simulink model "DTU_Topology_Rural"  (R2023b)
settings: Solver=ode4  StartTime=0.0  StopTime=stoptime  FixedStep=Ts  RelTol=1e-3
PreLoadFcn:
  | Ts=1e-4;load('RuralCase_11052022_12052022_Data_with_ParThreads_Final.mat');run('line_parameters.m');run('Grid_Parameters_3ph.m');
PostLoadFcn:
  | Ts=1e-4;load('RuralCase_11052022_12052022_Data_with_ParThreads_Final.mat');run('line_parameters.m');run('Grid_Parameters_3ph.m');
InitFcn:
  | Ts=1e-4;load('RuralCase_11052022_12052022_Data_with_ParThreads_Final.mat');run('line_parameters.m');run('Grid_Parameters_3ph.m');
StartFcn:
  | Ts=1e-4;load('RuralCase_11052022_12052022_Data_with_ParThreads_Final.mat');run('line_parameters.m');run('Grid_Parameters_3ph.m');
values from neighbouring files (symbols this model uses):
  datastart = 1    [Grid_Parameters_3ph.m]
  datastop = 21556    [Grid_Parameters_3ph.m]
  DTUsignconv = -1000    [Grid_Parameters_3ph.m]
  fnom = 50    [Grid_Parameters_3ph.m]    (also in line_parameters.m)
  line_param = struct()    [line_parameters.m]
  Time = cumsum([0;ones(stoptime,1)])    [Grid_Parameters_3ph.m]
  timestep_meas_data = 1    [Grid_Parameters_3ph.m]
  Vnom = 400    [Grid_Parameters_3ph.m]
undefined symbols (not defined in the file or in its folder): another_event_name, data, j, my_event_name, Newton, Raphson, t_factor
libraries: spsSeriesRLCBranchLib x126, spsGroundLib x71, spsThreePhaseSineGeneratorLib x42, spsControlledCurrentSourceLib x39, spsThreePhaseVIMeasurementLib x26, spsMeanLib x24, spsPowerLib x14, spsMutualInductanceLib x7, rtlab x3, powerlib_meascontrol x3, spsControlledVoltageSourceLib x3, spsThreePhaseSourceLib x1
(part 1 of 5)
Description:
  | Model of a simple control system for use iin training.
settings Model: VariantFading=off  Creator=Alex  LastModifiedBy=obus
settings SolverCC: AlgebraicLoopSolver=TrustRegion  AutoInsertRateTranBlk=on
settings DataIOCC: LimitDataPoints=on  SaveFormat=Array  SignalLoggingSaveFormat=ModelDataLogs  SaveOutput=off  SaveTime=off  ReturnWorkspaceOutputs=off  SignalLoggingName=sigsOut
settings OptimizationCC: BlockReduction=off  BooleanDataType=off  OptimizeBlockIOStorage=off  BufferReuse=off  GlobalBufferReuse=off  ExpressionFolding=off  LocalBlockOutputs=off  InitFltsAndDblsToZero=on  LifeSpan=inf  OptimizeDataStoreBuffers=off  BusAssignmentInplaceUpdate=off
settings DebuggingCC: SaveWithParameterizedLinksMsg=none  UnderspecifiedInitializationDetection=Classic  MergeDetectMultiDrivingBlocksExec=none  SignalResolutionControl=TryResolveAllWithWarning  MultiTaskDSMMsg=warning  MultiTaskCondExecSysMsg=none  FcnCallInpInsideContextMsg=warning  UnconnectedInputMsg=warning  UnconnectedOutputMsg=warning  UnconnectedLineMsg=warning  SFUnexpectedBacktrackingDiag=warning  SFNoUnconditionalDefaultTransitionDiag=warning  SFExecutionAtInitializationDiag=none  ArithmeticOperatorsInVariantConditions=warning
settings HardwareCC: ProdBitPerPointer=32  ProdBitPerSizeT=32  ProdBitPerPtrDiffT=32  ProdLargestAtomicFloat=None  ProdIntDivRoundTo=Undefined  ProdEndianess=Unspecified  ProdWordSize=32  ProdHWDeviceType=32-bit Generic  TargetUnknown=on
settings ModelReferenceCC: EnableRefExpFcnMdlSchedulingChecks=on  PropagateSignalLabelsOutOfModel=off
settings SFSimCC: SimUseLocalCustomCode=off  CustomCodeUndefinedFunction=UseInterfaceOnly
settings RTWCC: RTWUseLocalCustomCode=off  DLArmComputeVersion=19.05
settings CodeAppCC: StateflowObjectComments=on
settings GRTTargetCC: TargetFcnLib=ansi_tfl_tmw.mat  TargetLangStandard=C89/C90 (ANSI)  CombineOutputUpdateFcns=off  GRTInterface=on
settings ConfigComp: CovMetricSettings=dw  CovSaveCumulativeToWorkspaceVar=on  CovSaveSingleToWorkspaceVar=on  CovExternalEMLEnable=off

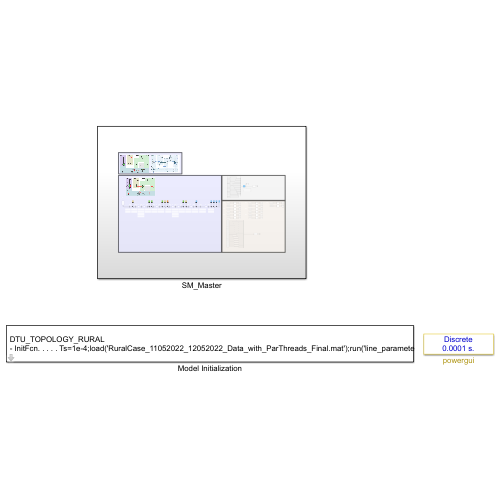
[thumbnail: Simulink's stored preview of the top-level diagram]
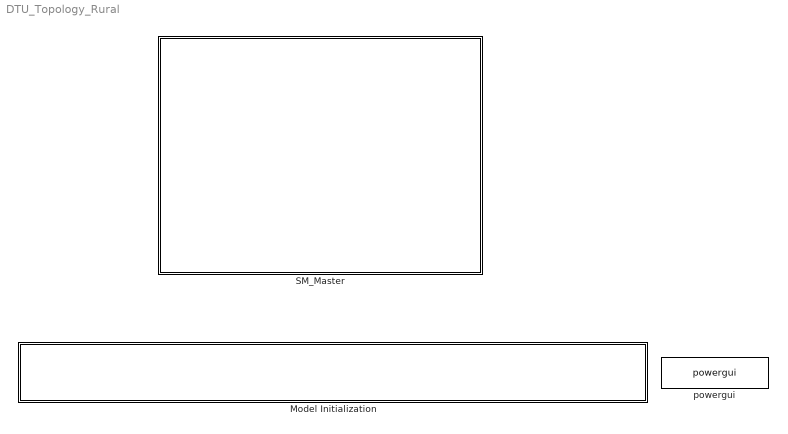
== system DTU_Topology_Rural ==
  Model Initialization : Subsystem  mask(Model Functions){InitFcnX=Ts=1e-4;load('RuralCase_11052022_12052022_Data_with_ParThreads_Final.mat');run('line_parameters.m');run('Grid_Parameters_3ph.m');, prel=on, posl=on, inif=on, strf=on}
      mask prompts: InitFcnX "Initialisation"; prel "Preload Function"; posl "PostLoad Function"; inif "InitFcn"; strf "StartFcn"
      mask init:
      | currentBlock = gcb;
      | root = bdroot(currentBlock);
      | 
      | if ~strcmp(get_param(root,'BlockDiagramType'),'library')
      |     if prel==1
      |         set_param(root, 'PreLoadFcn', InitFcnX);
      |     else
      |         set_param(root, 'PreLoadFcn', '');
      |     end
      |     if inif==1
      |         set_param(root, 'InitFcn', InitFcnX);
      |     else
      |         set_param(root, 'InitFcn', '');
      |     end
      |     if strf==1
      |         set_param(root, 'StartFcn', InitFcnX);
      |     else
      |         set_param(root, 'StartFcn', '');
      |     end
      |     if posl==1
      |         set_param(root, 'PostLoadFcn', InitFcnX);
      |     else
      |         set_param(root, 'PostLoadFcn', '');
      |     end
      | end
      | 
      | pos = get_param(currentBlock, 'Position');
      | width = pos(3) - pos(1); height = pos(4) - pos(2);
      | txt = [ upper(root) '\n' '- InitFcn. . . . . '  get_param(root, 'InitFcn') ];
      settings: CopyFcn=set_param(gcb,'LinkStatus','none')
      mask Display: text(5, height*0.5, txt, 'horizontalAlignment', 'left', 'verticalAlignment', 'middle') ;
  SM_Master : Subsystem
  powergui : sps_lib/powergui  Priority=2  SimulationMode=Discrete  SampleTime=Ts  frequency=60  Iterations=50  frequencyindice=50  Pbase=100e6  ErrMax=1e-4  UnitsV=V  UnitsW=kW  buscounter=0  FunctionMessages=off  echomessages=off  EnableUseOfTLC=off  CurrentSourceSwitches=off  DisableSnubberDevices=off  DisableRonSwitches=off  DisableVfSwitches=off  DisplayEquations=off  AutomaticDiscreteSolvers=off  SolverType=Tustin  Interpol=off  ExternalGateDelay=off  methode=off  Ts=0  x0status=steady  SPID=off  SwTol=0  HookPort=off  NonlinearTolerance=0  nMaxIteration=15  ContinueOnMaxIteration=off  RestoreLinks=warning  ResistiveCurrentMeasurement=off  Frange=logspace(0,3,50)  Ylog=off  Xlog=off  ShowGrid=off  save=off  variable=ZData  structure=0  ZoomFFT=on  StartTime=0.0  cycles=1  DisplayStyle=1  fundamental=60  FreqAxis=off  MaxFrequency=1000  frequencyindicesteady=1  RmsSteady=2  display=off

== system DTU_Topology_Rural/Model Initialization ==

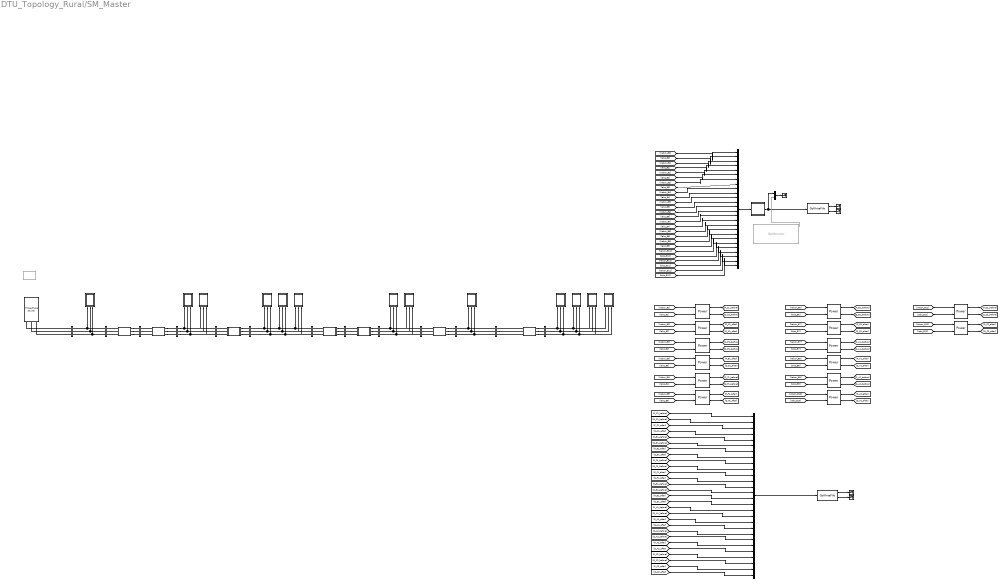
== system DTU_Topology_Rural/SM_Master ==
  note: 700m
  note: DTU SYSLAB Rural Topology
  note: Topology
  note: delta C1
  note: RT-Signals
  note: delta F1
  note: ΔP & ΔQ calculations
  note: delta E1
  note: Iabc_B0
  note: Vabcn_B0
  note: Vabcn_B1
  note: Iabc_B1
  note: Vabcn_B2
  note: Iabc_B2
  note: Vabcn_B3
  note: Iabc_B3
  note: Iabc_B4
  note: Vabcn_B4
  note: Iabc_B5
  note: Vabcn_B5
  note: Vabcn_B6
  note: Iabc_B6
  note: Iabc_B7
  note: Vabcn_B7
  note: Iabc_B8
  note: Vabcn_B8
  note: Vabcn_B9
  note: Iabc_B9
  note: Iabc_B10
  note: Vabcn_B10
  note: Vabcn_B12
  note: Iabc_B12
  note: delta A1
  note: delta A2
  note: delta B1
  note: delta C2
  note: 2:4
      | '117-2_Grid_phaseA_Voltage',
      | '117-2_Grid_phaseB_Voltage',
      | '117-2_Grid_phaseC_Voltage'
  note: 5:7
      | '117-2_Grid_phaseA_Current',
      | '117-2_Grid_phaseB_Current',
      | '117-2_Grid_phaseC_Current'
  note: 8:10
      | '117-2_Cable1_phaseA_Voltage',
      | '117-2_Cable1_phaseB_Voltage',
      | '117-2_Cable1_phaseC_Voltage'
  note: 11:13
      | '117-2_Cable1_phaseA_Current',
      | '117-2_Cable1_phaseB_Current',
      | '117-2_Cable1_phaseC_Current'
  note: 17:19
      | '319-3_C1 to 117-2_phaseA_Current',
      | '319-3_C1 to 117-2_phaseB_Current',
      | '319-3_C1 to 117-2_phaseC_Current'
  note: 14:16
      | '319-3_C1 to 117-2_phaseA_Voltage',
      | '319-3_C1 to 117-2_phaseB_Voltage',
      | '319-3_C1 to 117-2_phaseC_Voltage'
  note: same as 17:19
      | '319-3_E1 to 716-2_phaseA_Current',
      | '319-3_E1 to 716-2_phaseB_Current',
      | '319-3_E1 to 716-2_phaseC_Current'
  note: same as 14:16
      | '319-3_E1 to 716-2_phaseA_Voltage',
      | '319-3_E1 to 716-2_phaseB_Voltage',
      | '319-3_E1 to 716-2_phaseC_Voltage'
  note: 23:25
      | '716-2_CableE1_phaseA_Current',
      | '716-2_CableE1_phaseB_Current',
      | '716-2_CableE1_phaseC_Current'
  note: 20:22
      | '716-2_CableE1_phaseA_Voltage',
      | '716-2_CableE1_phaseB_Voltage',
      | '716-2_CableE1_phaseC_Voltage'
  note: 26:28
      | '716-2_Cable F1_phaseA_Voltage',
      | '716-2_Cable F1_phaseB_Voltage',
      | '716-2_Cable F1_phaseC_Voltage'
  note: 29:31
      | '716-2_Cable F1_phaseA_Current',
      | '716-2_Cable F1_phaseB_Current',
      | '716-2_Cable F1_phaseC_Current'
  note: 35:37
      | '715-2_CableF1_phaseA_Current',
      | '715-2_CableF1_phaseB_Current',
      | '715-2_CableF1_phaseC_Current'
  note: 32:34
      | '715-2_CableF1_phaseA_Voltage',
      | '715-2_CableF1_phaseB_Voltage',
      | '715-2_CableF1_phaseC_Voltage'
  note: 38:40
      | '715-2_CableB1_phaseA_Voltage',
      | '715-2_CableB1_phaseB_Voltage',
      | '715-2_CableB1_phaseC_Voltage'
  note: 41:43
      | '715-2_CableB1_phaseA_Current',
      | '715-2_CableB1_phaseB_Current',
      | '715-2_CableB1_phaseC_Current'
  note: 47:49
      | '319-3_B1 to 715-2_phaseA_Current',
      | '319-3_B1 to 715-2_phaseB_Current',
      | '319-3_B1 to 715-2_phaseC_Current'
  note: 44:46
      | '319-3_B1 to 715-2_phaseA_Voltage',
      | '319-3_B1 to 715-2_phaseB_Voltage',
      | '319-3_B1 to 715-2_phaseC_Voltage'
  note: same as 47:49
      | '319-3_A1 to 319-2_phaseA_Current',
      | '319-3_A1 to 319-2_phaseB_Current',
      | '319-3_A1 to 319-2_phaseC_Current'
  note: same as 44:46
      | '319-3_A1 to 319-2_phaseA_Voltage',
      | '319-3_A1 to 319-2_phaseB_Voltage',
      | '319-3_A1 to 319-2_phaseC_Voltage'
  note: 53:55
      | '319-2_Cable1_phaseA_Current',
      | '319-2_Cable1_phaseB_Current',
      | '319-2_Cable1_phaseC_Current'
  note: 50:52
      | '319-2_Cable1_phaseA_Voltage',
      | '319-2_Cable1_phaseB_Voltage',
      | '319-2_Cable1_phaseC_Voltage'
  note: 59:61
      | '319-2_Cable2_phaseA_Current',
      | '319-2_Cable2_phaseB_Current',
      | '319-2_Cable2_phaseC_Current'
  note: 56:58
      | '319-2_Cable2_phaseA_Voltage',
      | '319-2_Cable2_phaseB_Voltage',
      | '319-2_Cable2_phaseC_Voltage'
  note: 68:70
      | '319-3_C2 to 117-2_phaseA_Voltage',
      | '319-3_C2 to 117-2_phaseB_Voltage',
      | '319-3_C2 to 117-2_phaseC_Voltage'
  note: 71:73
      | '319-3_C2 to 117-2_phaseA_Current',
      | '319-3_C2 to 117-2_phaseB_Current',
      | '319-3_C2 to 117-2_phaseC_Current'
  note: 62:64
      | '319-3_A2 to 319-2_phaseA_Voltage',
      | '319-3_A2 to 319-2_phaseB_Voltage',
      | '319-3_A2 to 319-2_phaseC_Voltage'
  note: 65:67
      | '319-3_A2 to 319-2_phaseA_Current',
      | '319-3_A2 to 319-2_phaseB_Current',
      | '319-3_A2 to 319-2_phaseC_Current'
  note: 77:79
      | '117-2_Cable2_phaseA_Current',
      | '117-2_Cable2_phaseB_Current',
      | '117-2_Cable2_phaseC_Current'
  note: 74:76
      | '117-2_Cable2_phaseA_Voltage',
      | '117-2_Cable2_phaseB_Voltage',
      | '117-2_Cable2_phaseC_Voltage'
  note: 450m
  note: 330m
  note: 350m
  note: 25m
  note: 25m
  note: 700m
  note: Iabc_B11
  note: Vabcn_B11
  B0_n : spsThreePhaseVIMeasurementLib/Three-Phase V-I Measurement  VoltageMeasurement=phase-to-ground  SetLabelV=on  LabelV=Vabcn_B0  Vpu=off  VpuLL=off  CurrentMeasurement=yes  SetLabelI=on  LabelI=Iabc_B0  Ipu=off  Pbase=900e6  Vbase=400  OutputType=Complex  PhasorSimulation=off  PSBequivalent=0
  B10_n : spsThreePhaseVIMeasurementLib/Three-Phase V-I Measurement  VoltageMeasurement=phase-to-ground  SetLabelV=on  LabelV=Vabcn_B10  Vpu=off  VpuLL=off  CurrentMeasurement=yes  SetLabelI=on  LabelI=Iabc_B10  Ipu=off  Pbase=900e6  Vbase=400  OutputType=Complex  PhasorSimulation=off  PSBequivalent=0
  B11_n : spsThreePhaseVIMeasurementLib/Three-Phase V-I Measurement  VoltageMeasurement=phase-to-ground  SetLabelV=on  LabelV=Vabcn_B11  Vpu=off  VpuLL=off  CurrentMeasurement=yes  SetLabelI=on  LabelI=Iabc_B11  Ipu=off  Pbase=900e6  Vbase=400  OutputType=Complex  PhasorSimulation=off  PSBequivalent=0
  B12_n : spsThreePhaseVIMeasurementLib/Three-Phase V-I Measurement  VoltageMeasurement=phase-to-ground  SetLabelV=on  LabelV=Vabcn_B12  Vpu=off  VpuLL=off  CurrentMeasurement=yes  SetLabelI=on  LabelI=Iabc_B12  Ipu=off  Pbase=900e6  Vbase=400  OutputType=Complex  PhasorSimulation=off  PSBequivalent=0
  B1_n : spsThreePhaseVIMeasurementLib/Three-Phase V-I Measurement  VoltageMeasurement=phase-to-ground  SetLabelV=on  LabelV=Vabcn_B1  Vpu=off  VpuLL=off  CurrentMeasurement=yes  SetLabelI=on  LabelI=Iabc_B1  Ipu=off  Pbase=900e6  Vbase=400  OutputType=Complex  PhasorSimulation=off  PSBequivalent=0
  B2_n : spsThreePhaseVIMeasurementLib/Three-Phase V-I Measurement  VoltageMeasurement=phase-to-ground  SetLabelV=on  LabelV=Vabcn_B2  Vpu=off  VpuLL=off  CurrentMeasurement=yes  SetLabelI=on  LabelI=Iabc_B2  Ipu=off  Pbase=900e6  Vbase=400  OutputType=Complex  PhasorSimulation=off  PSBequivalent=0
  B3_n : spsThreePhaseVIMeasurementLib/Three-Phase V-I Measurement  VoltageMeasurement=phase-to-ground  SetLabelV=on  LabelV=Vabcn_B3  Vpu=off  VpuLL=off  CurrentMeasurement=yes  SetLabelI=on  LabelI=Iabc_B3  Ipu=off  Pbase=900e6  Vbase=400  OutputType=Complex  PhasorSimulation=off  PSBequivalent=0
  B4_n : spsThreePhaseVIMeasurementLib/Three-Phase V-I Measurement  VoltageMeasurement=phase-to-ground  SetLabelV=on  LabelV=Vabcn_B4  Vpu=off  VpuLL=off  CurrentMeasurement=yes  SetLabelI=on  LabelI=Iabc_B4  Ipu=off  Pbase=900e6  Vbase=400  OutputType=Complex  PhasorSimulation=off  PSBequivalent=0
  B5_n : spsThreePhaseVIMeasurementLib/Three-Phase V-I Measurement  VoltageMeasurement=phase-to-ground  SetLabelV=on  LabelV=Vabcn_B5  Vpu=off  VpuLL=off  CurrentMeasurement=yes  SetLabelI=on  LabelI=Iabc_B5  Ipu=off  Pbase=900e6  Vbase=400  OutputType=Complex  PhasorSimulation=off  PSBequivalent=0
  B6_n : spsThreePhaseVIMeasurementLib/Three-Phase V-I Measurement  VoltageMeasurement=phase-to-ground  SetLabelV=on  LabelV=Vabcn_B6  Vpu=off  VpuLL=off  CurrentMeasurement=yes  SetLabelI=on  LabelI=Iabc_B6  Ipu=off  Pbase=900e6  Vbase=400  OutputType=Complex  PhasorSimulation=off  PSBequivalent=0
  B7_n : spsThreePhaseVIMeasurementLib/Three-Phase V-I Measurement  VoltageMeasurement=phase-to-ground  SetLabelV=on  LabelV=Vabcn_B7  Vpu=off  VpuLL=off  CurrentMeasurement=yes  SetLabelI=on  LabelI=Iabc_B7  Ipu=off  Pbase=900e6  Vbase=400  OutputType=Complex  PhasorSimulation=off  PSBequivalent=0
  B8_n : spsThreePhaseVIMeasurementLib/Three-Phase V-I Measurement  VoltageMeasurement=phase-to-ground  SetLabelV=on  LabelV=Vabcn_B8  Vpu=off  VpuLL=off  CurrentMeasurement=yes  SetLabelI=on  LabelI=Iabc_B8  Ipu=off  Pbase=900e6  Vbase=400  OutputType=Complex  PhasorSimulation=off  PSBequivalent=0
  B9_n : spsThreePhaseVIMeasurementLib/Three-Phase V-I Measurement  VoltageMeasurement=phase-to-ground  SetLabelV=on  LabelV=Vabcn_B9  Vpu=off  VpuLL=off  CurrentMeasurement=yes  SetLabelI=on  LabelI=Iabc_B9  Ipu=off  Pbase=900e6  Vbase=400  OutputType=Complex  PhasorSimulation=off  PSBequivalent=0
  Cable A1 No parallel cap : Subsystem  mask(ZHAW_Config){fNom=fnom, length=line_param.A1.length}
      mask prompts: fNom "Nominal frequency (Hz)"; length "Length (km)"
      mask Display:
      | patch([20 20 80 80], [0 20 20 0])
      | patch([0 0 20 20], [7 13 13 7])
      | patch([80 80 100 100], [7 13 13 7])
      | 
      | patch([20 20 80 80], [40 60 60 40])
      | patch([0 0 20 20], [47 53 53 47])
      | patch([80 80 100 100], [47 53 53 47])
      | 
      | patch([20 20 80 80], [80 100 100 80])
      | patch([0 0 20 20], [87 93 93 87])
      | patch([80 80 100 100], [87 93 93 87])
  Cable A2 No parallel cap : Subsystem  mask(ZHAW_Config){fNom=fnom, length=line_param.A2.length}
      mask prompts: fNom "Nominal frequency (Hz)"; length "Length (km)"
      mask Display:
      | patch([20 20 80 80], [0 20 20 0])
      | patch([0 0 20 20], [7 13 13 7])
      | patch([80 80 100 100], [7 13 13 7])
      | 
      | patch([20 20 80 80], [40 60 60 40])
      | patch([0 0 20 20], [47 53 53 47])
      | patch([80 80 100 100], [47 53 53 47])
      | 
      | patch([20 20 80 80], [80 100 100 80])
      | patch([0 0 20 20], [87 93 93 87])
      | patch([80 80 100 100], [87 93 93 87])
  Cable B1 No parallel cap : Subsystem  mask(ZHAW_Config){fNom=fnom, length=line_param.B1.length}
      mask prompts: fNom "Nominal frequency (Hz)"; length "Length (km)"
      mask Display:
      | patch([20 20 80 80], [0 20 20 0])
      | patch([0 0 20 20], [7 13 13 7])
      | patch([80 80 100 100], [7 13 13 7])
      | 
      | patch([20 20 80 80], [40 60 60 40])
      | patch([0 0 20 20], [47 53 53 47])
      | patch([80 80 100 100], [47 53 53 47])
      | 
      | patch([20 20 80 80], [80 100 100 80])
      | patch([0 0 20 20], [87 93 93 87])
      | patch([80 80 100 100], [87 93 93 87])
  Cable C1 No parallel cap : Subsystem  mask(ZHAW_Config){fNom=fnom, length=line_param.C1.length}
      mask prompts: fNom "Nominal frequency (Hz)"; length "Length (km)"
      mask Display:
      | patch([20 20 80 80], [0 20 20 0])
      | patch([0 0 20 20], [7 13 13 7])
      | patch([80 80 100 100], [7 13 13 7])
      | 
      | patch([20 20 80 80], [40 60 60 40])
      | patch([0 0 20 20], [47 53 53 47])
      | patch([80 80 100 100], [47 53 53 47])
      | 
      | patch([20 20 80 80], [80 100 100 80])
      | patch([0 0 20 20], [87 93 93 87])
      | patch([80 80 100 100], [87 93 93 87])
  Cable C2 No parallel cap : Subsystem  mask(ZHAW_Config){fNom=fnom, length=line_param.C2.length}
      mask prompts: fNom "Nominal frequency (Hz)"; length "Length (km)"
      mask Display:
      | patch([20 20 80 80], [0 20 20 0])
      | patch([0 0 20 20], [7 13 13 7])
      | patch([80 80 100 100], [7 13 13 7])
      | 
      | patch([20 20 80 80], [40 60 60 40])
      | patch([0 0 20 20], [47 53 53 47])
      | patch([80 80 100 100], [47 53 53 47])
      | 
      | patch([20 20 80 80], [80 100 100 80])
      | patch([0 0 20 20], [87 93 93 87])
      | patch([80 80 100 100], [87 93 93 87])
  Cable E1 No parallel cap : Subsystem  mask(ZHAW_Config){fNom=fnom, length=line_param.E1.length}
      mask prompts: fNom "Nominal frequency (Hz)"; length "Length (km)"
      mask Display:
      | patch([20 20 80 80], [0 20 20 0])
      | patch([0 0 20 20], [7 13 13 7])
      | patch([80 80 100 100], [7 13 13 7])
      | 
      | patch([20 20 80 80], [40 60 60 40])
      | patch([0 0 20 20], [47 53 53 47])
      | patch([80 80 100 100], [47 53 53 47])
      | 
      | patch([20 20 80 80], [80 100 100 80])
      | patch([0 0 20 20], [87 93 93 87])
      | patch([80 80 100 100], [87 93 93 87])
  Cable F1 No parallel cap : Subsystem  mask(ZHAW_Config){fNom=fnom, length=line_param.F1.length}
      mask prompts: fNom "Nominal frequency (Hz)"; length "Length (km)"
      mask Display:
      | patch([20 20 80 80], [0 20 20 0])
      | patch([0 0 20 20], [7 13 13 7])
      | patch([80 80 100 100], [7 13 13 7])
      | 
      | patch([20 20 80 80], [40 60 60 40])
      | patch([0 0 20 20], [47 53 53 47])
      | patch([80 80 100 100], [47 53 53 47])
      | 
      | patch([20 20 80 80], [80 100 100 80])
      | patch([0 0 20 20], [87 93 93 87])
      | patch([80 80 100 100], [87 93 93 87])
  External Grid 400V : spsThreePhaseSourceLib/Three-Phase Source  InternalConnection=Yg  VoltagePhases=off  Voltage=400  PhaseAngle=0  Voltage_phases=[400 400 400]/sqrt(3)*1.00006  PhaseAngles_phases=[0 -120 +120]  Frequency=50  NonIdealSource=on  SpecifyImpedance=on  Resistance=400^2/10e6/10  Inductance=400^2/10e6/(2*pi*50)  ShortCircuitLevel=60e6  BaseVoltage=400  XRratio=1/0.1  BusType=swing  Pref=0  Qref=0  Prefabc=[10e3, 10e3, 10e3]  Qrefabc=[0, 0, 0]  Qmin=-Inf  Qmax=Inf
  Mux2 : Mux  Inputs=2
  Mux3 : Mux  Inputs=3*ones(1,26)
  Mux5 : Mux  Inputs=3 * ones(1,28)
  OpMonitor : rtlab/Monitoring/OpMonitor  Commented=on  compute_time=on  real_step=on  idle_time=on  nb_overruns=on  user_time=off  user_name=my_event_name,another_event_name
      settings: SourceProductName=RT-LAB
  OpWriteFile : rtlab/DataLogging/OpWriteFile  Static_File=on  varname=DTU_Rural_Case_x_UI  Filename=DTU_Rural_Case_x_UI.mat  rtpath='./'  nrtpath='.\'  Acq_Group=26  file_size=[500e6]  write_offline=on  Sim_Mode=off  Nb_Samples=stoptime  Buffer_size=1000000
      settings: SourceProductName=RT-LAB  Decimation=10000
  OpWriteFile1 : rtlab/DataLogging/OpWriteFile  Static_File=on  varname=DTU_Rural_Case_x_PQ  Filename=DTU_Rural_Case_x_PQ.mat  rtpath='./'  nrtpath='.\'  Acq_Group=27  file_size=[500e6]  write_offline=on  Sim_Mode=off  Nb_Samples=stoptime  Buffer_size=1000000
      settings: SourceProductName=RT-LAB  Decimation=10000
  Power{,1..13} (14 alike) : spsPowerLib/Power  Freq=50  Vinit=[1, 0]  Iinit=[1, 0]  Ts=0
  Terminator{,1..4} (5 alike) : Terminator
  TrueRMS 1 : Subsystem  AncestorBlock=powerlib_meascontrol/Measurements/RMS/TrueRMS
  Uncontrollable EVSE 4 : Subsystem
  Uncontrollable EVSE 5 : Subsystem
  Uncontrollable EVSE 6 : Subsystem
  Uncontrollable EVSE 7 : Subsystem
  Uncontrollable EVSE V2G & EVSE SYSLAB : Subsystem
  Uncontrollable PV 117 : Subsystem
  Uncontrollable PV 319 : Subsystem
  Uncontrollable PV 715 : Subsystem
  Uncontrollable Load (Dump load) : Subsystem
  Uncontrollable Load (Flexhouse 2) : Subsystem
  Uncontrollable Load (Flexhouse 3) : Subsystem
  Uncontrollable Load (Flexhouse) : Subsystem
  Uncontrollable Wind Turbine (Gaia) : Subsystem
  Voltage Source : Subsystem  Commented=on
  wires:
  Power8/2 -> [Q_E1_before]
  TrueRMS 1/1(RMS) -> Mux2/1, OpWriteFile/1
  Power11/2 -> [Q_F1_after]
  Power10/2 -> [Q_F1_before]
  [Vabcn_B1] -> Power/1
  OpWriteFile/1 -> Terminator/1
  Power/1 -> [P_C1_before]
  [Vabcn_B2] -> Power1/1
  Power9/2 -> [Q_E1_after]
  [Iabc_B4] -> Power10/2
  Power10/1 -> [P_F1_before]
  OpWriteFile1/1 -> Terminator3/1
  [Vabcn_B5] -> Power11/1
  Power11/1 -> [P_F1_after]
  [Vabcn_B4] -> Power10/1
  [Iabc_B2] -> Power8/2
  Power8/1 -> [P_E1_before]
  [Iabc_B3] -> Power9/2
  [Iabc_B5] -> Power11/2
  OpWriteFile/2 -> Terminator1/1
  Mux5/1 -> OpWriteFile1/1
  Power9/1 -> [P_E1_after]
  Power/2 -> [Q_C1_before]
  [Iabc_B1] -> Power/2
  [Iabc_B2] -> Power1/2
  Power1/2 -> [Q_C1_after]
  OpWriteFile1/2 -> Terminator4/1
  [Vabcn_B2] -> Power8/1
  OpMonitor/1 -> Mux2/2
  [Vabcn_B3] -> Power9/1
  Mux2/1 -> Terminator2/1
  Power1/1 -> [P_C1_after]
  Mux3/1 -> TrueRMS 1/1(In)
  [Vabcn_B0] -> Mux3/1
  [Iabc_B0] -> Mux3/2
  [Vabcn_B1] -> Mux3/3
  [Iabc_B1] -> Mux3/4
  [Vabcn_B2] -> Mux3/5
  [Iabc_B2] -> Mux3/6
  [Vabcn_B3] -> Mux3/7
  [Iabc_B3] -> Mux3/8
  [Vabcn_B4] -> Mux3/9
  [Iabc_B4] -> Mux3/10
  [Vabcn_B5] -> Mux3/11
  [Iabc_B5] -> Mux3/12
  [Vabcn_B6] -> Mux3/13
  [Iabc_B6] -> Mux3/14
  [Vabcn_B7] -> Mux3/15
  [Iabc_B7] -> Mux3/16
  [Vabcn_B8] -> Mux3/17
  [Iabc_B8] -> Mux3/18
  [Vabcn_B9] -> Mux3/19
  [Iabc_B9] -> Mux3/20
  [Vabcn_B10] -> Mux3/21
  [Iabc_B10] -> Mux3/22
  [Vabcn_B11] -> Mux3/23
  [Iabc_B11] -> Mux3/24
  Power3/1 -> [P_B1_after]
  Power4/2 -> [Q_A2_before]
  Power5/2 -> [Q_A2_after]
  Power6/2 -> [Q_A1_before]
  [Vabcn_B8] -> Power7/1
  [Vabcn_B7] -> Power6/1
  [Iabc_B6] -> Power2/2
  [Vabcn_B6] -> Power2/1
  Power7/1 -> [P_A1_after]
  Power2/1 -> [P_B1_before]
  Power3/2 -> [Q_B1_after]
  Power2/2 -> [Q_B1_before]
  [Iabc_B10] -> Power5/2
  [Iabc_B8] -> Power7/2
  [Iabc_B7] -> Power6/2
  [Iabc_B7] -> Power3/2
  [Vabcn_B9] -> Power4/1
  Power4/1 -> [P_A2_before]
  [Vabcn_B10] -> Power5/1
  [Vabcn_B7] -> Power3/1
  [Iabc_B9] -> Power4/2
  Power6/1 -> [P_A1_before]
  Power7/2 -> [Q_A1_after]
  Power5/1 -> [P_A2_after]
  Power13/2 -> [Q_C2_after]
  Power12/2 -> [Q_C2_before]
  [Iabc_B12] -> Power13/2
  [Iabc_B11] -> Power12/2
  [Vabcn_B11] -> Power12/1
  Power12/1 -> [P_C2_before]
  Power13/1 -> [P_C2_after]
  [Vabcn_B12] -> Power13/1
  [P_C1_before] -> Mux5/1
  [Q_C1_before] -> Mux5/2
  [P_C1_after] -> Mux5/3
  [Q_C1_after] -> Mux5/4
  [P_E1_before] -> Mux5/5
  [Q_E1_before] -> Mux5/6
  [P_E1_after] -> Mux5/7
  [Q_E1_after] -> Mux5/8
  [P_F1_before] -> Mux5/9
  [Q_F1_before] -> Mux5/10
  [P_F1_after] -> Mux5/11
  [Q_F1_after] -> Mux5/12
  [P_B1_before] -> Mux5/13
  [Q_B1_before] -> Mux5/14
  [P_B1_after] -> Mux5/15
  [Q_B1_after] -> Mux5/16
  [P_A1_before] -> Mux5/17
  [Q_A1_before] -> Mux5/18
  [P_A1_after] -> Mux5/19
  [Q_A1_after] -> Mux5/20
  [P_A2_before] -> Mux5/21
  [Q_A2_before] -> Mux5/22
  [P_A2_after] -> Mux5/23
  [Q_A2_after] -> Mux5/24
  [P_C2_before] -> Mux5/25
  [Q_C2_before] -> Mux5/26
  [P_C2_after] -> Mux5/27
  [Q_C2_after] -> Mux5/28
  [Vabcn_B12] -> Mux3/25
  [Iabc_B12] -> Mux3/26
  connections:
  Uncontrollable PV 117/RConn3 -- B1_n/LConn3 -- B0_n/RConn3
  Uncontrollable PV 117/RConn2 -- B1_n/LConn2 -- B0_n/RConn2
  Uncontrollable PV 117/RConn1 -- B1_n/LConn1 -- B0_n/RConn1
  Cable C1 No parallel cap/RConn2 -- B2_n/LConn2
  Cable C1 No parallel cap/LConn1 -- B1_n/RConn1
  Cable C1 No parallel cap/RConn1 -- B2_n/LConn1
  Cable C1 No parallel cap/RConn3 -- B2_n/LConn3
  Cable C1 No parallel cap/LConn2 -- B1_n/RConn2
  Cable C1 No parallel cap/LConn3 -- B1_n/RConn3
  Cable E1 No parallel cap/LConn1 -- B2_n/RConn1
  Cable E1 No parallel cap/LConn2 -- B2_n/RConn2
  Cable E1 No parallel cap/LConn3 -- B2_n/RConn3
  Uncontrollable Load (Flexhouse 2)/RConn1 -- B3_n/RConn1 -- B4_n/LConn1 -- Uncontrollable Load (Flexhouse 3)/RConn1
  B4_n/LConn2 -- Uncontrollable Load (Flexhouse 3)/RConn2 -- B3_n/RConn2 -- Uncontrollable Load (Flexhouse 2)/RConn2
  Uncontrollable Load (Flexhouse 2)/RConn3 -- B3_n/RConn3 -- B4_n/LConn3 -- Uncontrollable Load (Flexhouse 3)/RConn3
  Cable F1 No parallel cap/LConn1 -- B4_n/RConn1
  Cable F1 No parallel cap/LConn2 -- B4_n/RConn2
  Cable F1 No parallel cap/LConn3 -- B4_n/RConn3
  Cable F1 No parallel cap/RConn1 -- B5_n/LConn1
  Cable F1 No parallel cap/RConn2 -- B5_n/LConn2
  Cable F1 No parallel cap/RConn3 -- B5_n/LConn3
  Uncontrollable Load (Flexhouse)/RConn1 -- B5_n/RConn1 -- B6_n/LConn1 -- Uncontrollable Wind Turbine (Gaia)/RConn1 -- Uncontrollable PV 715/RConn1
  Uncontrollable Load (Flexhouse)/RConn2 -- B5_n/RConn2 -- B6_n/LConn2 -- Uncontrollable Wind Turbine (Gaia)/RConn2 -- Uncontrollable PV 715/RConn2
  Uncontrollable Load (Flexhouse)/RConn3 -- B5_n/RConn3 -- B6_n/LConn3 -- Uncontrollable Wind Turbine (Gaia)/RConn3 -- Uncontrollable PV 715/RConn3
  Cable B1 No parallel cap/LConn1 -- B6_n/RConn1
  Cable B1 No parallel cap/LConn2 -- B6_n/RConn2
  Cable B1 No parallel cap/LConn3 -- B6_n/RConn3
  Cable B1 No parallel cap/RConn1 -- B7_n/LConn1
  Cable B1 No parallel cap/RConn2 -- B7_n/LConn2
  Cable B1 No parallel cap/RConn3 -- B7_n/LConn3
  Cable A1 No parallel cap/LConn1 -- B7_n/RConn1
  Cable A1 No parallel cap/LConn2 -- B7_n/RConn2
  Cable A1 No parallel cap/LConn3 -- B7_n/RConn3
  Cable A1 No parallel cap/RConn1 -- B8_n/LConn1
  Cable A1 No parallel cap/RConn2 -- B8_n/LConn2
  Cable A1 No parallel cap/RConn3 -- B8_n/LConn3
  B9_n/LConn1 -- Uncontrollable PV 319/RConn1 -- B8_n/RConn1 -- Uncontrollable Load (Dump load)/RConn1
  Uncontrollable Load (Dump load)/RConn2 -- B8_n/RConn2 -- B9_n/LConn2 -- Uncontrollable PV 319/RConn2
  B9_n/LConn3 -- Uncontrollable PV 319/RConn3 -- B8_n/RConn3 -- Uncontrollable Load (Dump load)/RConn3
  Cable A2 No parallel cap/RConn1 -- B10_n/LConn1
  Cable A2 No parallel cap/RConn2 -- B10_n/LConn2
  Cable A2 No parallel cap/RConn3 -- B10_n/LConn3
  Uncontrollable EVSE V2G & EVSE SYSLAB/RConn1 -- B11_n/LConn1 -- B10_n/RConn1
  Uncontrollable EVSE V2G & EVSE SYSLAB/RConn2 -- B11_n/LConn2 -- B10_n/RConn2
  Uncontrollable EVSE V2G & EVSE SYSLAB/RConn3 -- B11_n/LConn3 -- B10_n/RConn3
  Cable C2 No parallel cap/RConn1 -- B12_n/LConn1
  Cable C2 No parallel cap/RConn2 -- B12_n/LConn2
  Cable C2 No parallel cap/RConn3 -- B12_n/LConn3
  Uncontrollable EVSE 4/RConn1 -- Uncontrollable EVSE 7/RConn1 -- Uncontrollable EVSE 6/RConn1 -- Uncontrollable EVSE 5/RConn1 -- B12_n/RConn1
  Uncontrollable EVSE 4/RConn2 -- Uncontrollable EVSE 7/RConn2 -- Uncontrollable EVSE 6/RConn2 -- Uncontrollable EVSE 5/RConn2 -- B12_n/RConn2
  Uncontrollable EVSE 4/RConn3 -- Uncontrollable EVSE 7/RConn3 -- Uncontrollable EVSE 6/RConn3 -- Uncontrollable EVSE 5/RConn3 -- B12_n/RConn3
  Cable A2 No parallel cap/LConn1 -- B9_n/RConn1
  Cable A2 No parallel cap/LConn2 -- B9_n/RConn2
  Cable A2 No parallel cap/LConn3 -- B9_n/RConn3
  Cable E1 No parallel cap/RConn1 -- B3_n/LConn1
  Cable E1 No parallel cap/RConn2 -- B3_n/LConn2
  Cable E1 No parallel cap/RConn3 -- B3_n/LConn3
  Cable C2 No parallel cap/LConn1 -- B11_n/RConn1
  B11_n/RConn2 -- Cable C2 No parallel cap/LConn2
  Cable C2 No parallel cap/LConn3 -- B11_n/RConn3
  B0_n/LConn1 -- External Grid 400V/RConn1
  B0_n/LConn2 -- External Grid 400V/RConn2
  B0_n/LConn3 -- External Grid 400V/RConn3

== system DTU_Topology_Rural/SM_Master/Cable A1 No parallel cap ==
  Config301 : spsMutualInductanceLib/Mutual Inductance  LConnTagsString=a|b|c  RConnTagsString=A|B|C  TypeOfMutual=Generalized mutual inductance  NumberOfWindings=3  SelfImpedance1=[1.1 1.1e-03]  SelfImpedance2=[ 1.1 1.1e-03]  ThreeWindings=on  SelfImpedance3=[ 1.1 1.1e-03]  MutualImpedance=[1.0 1.0e-03]  InductanceMatrix=[line_param.A1.Ls line_param.A1.Lm line_param.A1.Lm ; line_param.A1.Lm line_param.A1.Ls line_param.A1.Lm ; line_param.A1.Lm line_param.A1.Lm line_param.A1.Ls]  ResistanceMatrix=[line_param.A1.Rs line_param.A1.Rm line_param.A1.Rm ; line_param.A1.Rm line_param.A1.Rs line_param.A1.Rm ; line_param.A1.Rm line_param.A1.Rm line_param.A1.Rs]  Measurements=None
      settings: LibrarySourceBlock=sps_lib/Passives/Mutual Inductance
  Ground{,1..5} (6 alike) : spsGroundLib/Ground  LConnTagsString=a
  Series RLC Branch{,1..5} (6 alike) : spsSeriesRLCBranchLib/Series RLC Branch  LConnTagsString=__new0  RConnTagsString=__new0  BranchType=C  Resistance=1  Inductance=1e-3  SetiL0=off  InitialCurrent=0  Capacitance=line_param.A1.Cg / 2  Setx0=off  InitialVoltage=0  Measurements=None
  Series RLC Branch{6..11} (6 alike) : spsSeriesRLCBranchLib/Series RLC Branch  Commented=on  LConnTagsString=__new0  RConnTagsString=__new0  BranchType=C  Resistance=1  Inductance=1e-3  SetiL0=off  InitialCurrent=0  Capacitance=line_param.A1.Cp / 2  Setx0=off  InitialVoltage=0  Measurements=None
  a : PMIOPort  Tag=PMCPort  Side=Left
  b : PMIOPort  Tag=PMCPort  Port=2  Side=Left
  c : PMIOPort  Tag=PMCPort  Port=3  Side=Left
  "a " : PMIOPort  Tag=PMCPort  Port=4  Side=Right
  "b " : PMIOPort  Tag=PMCPort  Port=5  Side=Right
  "c " : PMIOPort  Tag=PMCPort  Port=6  Side=Right
  connections:
  Series RLC Branch5/RConn1 -- Ground5/LConn1
  Series RLC Branch4/RConn1 -- Ground4/LConn1
  Series RLC Branch3/RConn1 -- Ground3/LConn1
  Series RLC Branch2/RConn1 -- Ground2/LConn1
  Series RLC Branch1/RConn1 -- Ground1/LConn1
  Series RLC Branch/RConn1 -- Ground/LConn1
  Series RLC Branch/LConn1 -- Config301/RConn3 -- Series RLC Branch8/RConn1 -- "c "/RConn1 -- Series RLC Branch6/RConn1
  Series RLC Branch1/LConn1 -- Config301/RConn2 -- Series RLC Branch7/RConn1 -- Series RLC Branch6/LConn1 -- "b "/RConn1
  Series RLC Branch2/LConn1 -- Config301/RConn1 -- Series RLC Branch8/LConn1 -- "a "/RConn1 -- Series RLC Branch7/LConn1
  Series RLC Branch5/LConn1 -- Config301/LConn3 -- Series RLC Branch11/RConn1 -- c/RConn1 -- Series RLC Branch10/RConn1
  Series RLC Branch4/LConn1 -- Config301/LConn2 -- Series RLC Branch10/LConn1 -- Series RLC Branch9/RConn1 -- b/RConn1
  Series RLC Branch3/LConn1 -- Config301/LConn1 -- Series RLC Branch11/LConn1 -- a/RConn1 -- Series RLC Branch9/LConn1

== system DTU_Topology_Rural/SM_Master/Cable A2 No parallel cap ==
  Config301 : spsMutualInductanceLib/Mutual Inductance  LConnTagsString=a|b|c  RConnTagsString=A|B|C  TypeOfMutual=Generalized mutual inductance  NumberOfWindings=3  SelfImpedance1=[1.1 1.1e-03]  SelfImpedance2=[ 1.1 1.1e-03]  ThreeWindings=on  SelfImpedance3=[ 1.1 1.1e-03]  MutualImpedance=[1.0 1.0e-03]  InductanceMatrix=[line_param.A2.Ls line_param.A2.Lm line_param.A2.Lm ; line_param.A2.Lm line_param.A2.Ls line_param.A2.Lm ; line_param.A2.Lm line_param.A2.Lm line_param.A2.Ls]  ResistanceMatrix=[line_param.A2.Rs line_param.A2.Rm line_param.A2.Rm ; line_param.A2.Rm line_param.A2.Rs line_param.A2.Rm ; line_param.A2.Rm line_param.A2.Rm line_param.A2.Rs]  Measurements=None
      settings: LibrarySourceBlock=sps_lib/Passives/Mutual Inductance
  Ground{,1..5} (6 alike) : spsGroundLib/Ground  LConnTagsString=a
  Series RLC Branch{,1..5} (6 alike) : spsSeriesRLCBranchLib/Series RLC Branch  LConnTagsString=__new0  RConnTagsString=__new0  BranchType=C  Resistance=1  Inductance=1e-3  SetiL0=off  InitialCurrent=0  Capacitance=line_param.A2.Cg / 2  Setx0=off  InitialVoltage=0  Measurements=None
  Series RLC Branch{6..11} (6 alike) : spsSeriesRLCBranchLib/Series RLC Branch  Commented=on  LConnTagsString=__new0  RConnTagsString=__new0  BranchType=C  Resistance=1  Inductance=1e-3  SetiL0=off  InitialCurrent=0  Capacitance=line_param.A2.Cp / 2  Setx0=off  InitialVoltage=0  Measurements=None
  a : PMIOPort  Tag=PMCPort  Side=Left
  b : PMIOPort  Tag=PMCPort  Port=2  Side=Left
  c : PMIOPort  Tag=PMCPort  Port=3  Side=Left
  "a " : PMIOPort  Tag=PMCPort  Port=4  Side=Right
  "b " : PMIOPort  Tag=PMCPort  Port=5  Side=Right
  "c " : PMIOPort  Tag=PMCPort  Port=6  Side=Right
  connections:
  Series RLC Branch5/RConn1 -- Ground5/LConn1
  Series RLC Branch4/RConn1 -- Ground4/LConn1
  Series RLC Branch3/RConn1 -- Ground3/LConn1
  Series RLC Branch2/RConn1 -- Ground2/LConn1
  Series RLC Branch1/RConn1 -- Ground1/LConn1
  Series RLC Branch/RConn1 -- Ground/LConn1
  Series RLC Branch/LConn1 -- Config301/RConn3 -- Series RLC Branch8/RConn1 -- "c "/RConn1 -- Series RLC Branch6/RConn1
  Series RLC Branch1/LConn1 -- Config301/RConn2 -- Series RLC Branch7/RConn1 -- Series RLC Branch6/LConn1 -- "b "/RConn1
  Series RLC Branch2/LConn1 -- Config301/RConn1 -- Series RLC Branch8/LConn1 -- "a "/RConn1 -- Series RLC Branch7/LConn1
  Series RLC Branch5/LConn1 -- Config301/LConn3 -- Series RLC Branch11/RConn1 -- c/RConn1 -- Series RLC Branch10/RConn1
  Series RLC Branch4/LConn1 -- Config301/LConn2 -- Series RLC Branch10/LConn1 -- Series RLC Branch9/RConn1 -- b/RConn1
  Series RLC Branch3/LConn1 -- Config301/LConn1 -- Series RLC Branch11/LConn1 -- a/RConn1 -- Series RLC Branch9/LConn1

== system DTU_Topology_Rural/SM_Master/Cable B1 No parallel cap ==
  Config301 : spsMutualInductanceLib/Mutual Inductance  LConnTagsString=a|b|c  RConnTagsString=A|B|C  TypeOfMutual=Generalized mutual inductance  NumberOfWindings=3  SelfImpedance1=[1.1 1.1e-03]  SelfImpedance2=[ 1.1 1.1e-03]  ThreeWindings=on  SelfImpedance3=[ 1.1 1.1e-03]  MutualImpedance=[1.0 1.0e-03]  InductanceMatrix=[line_param.B1.Ls line_param.B1.Lm line_param.B1.Lm ; line_param.B1.Lm line_param.B1.Ls line_param.B1.Lm ; line_param.B1.Lm line_param.B1.Lm line_param.B1.Ls]  ResistanceMatrix=[line_param.B1.Rs line_param.B1.Rm line_param.B1.Rm ; line_param.B1.Rm line_param.B1.Rs line_param.B1.Rm ; line_param.B1.Rm line_param.B1.Rm line_param.B1.Rs]  Measurements=None
      settings: LibrarySourceBlock=sps_lib/Passives/Mutual Inductance
  Ground{,1..5} (6 alike) : spsGroundLib/Ground  LConnTagsString=a
  Series RLC Branch{,1..5} (6 alike) : spsSeriesRLCBranchLib/Series RLC Branch  LConnTagsString=__new0  RConnTagsString=__new0  BranchType=C  Resistance=1  Inductance=1e-3  SetiL0=off  InitialCurrent=0  Capacitance=line_param.B1.Cg / 2  Setx0=off  InitialVoltage=0  Measurements=None
  Series RLC Branch{6..11} (6 alike) : spsSeriesRLCBranchLib/Series RLC Branch  Commented=on  LConnTagsString=__new0  RConnTagsString=__new0  BranchType=C  Resistance=1  Inductance=1e-3  SetiL0=off  InitialCurrent=0  Capacitance=line_param.B1.Cp / 2  Setx0=off  InitialVoltage=0  Measurements=None
  a : PMIOPort  Tag=PMCPort  Side=Left
  b : PMIOPort  Tag=PMCPort  Port=2  Side=Left
  c : PMIOPort  Tag=PMCPort  Port=3  Side=Left
  "a " : PMIOPort  Tag=PMCPort  Port=4  Side=Right
  "b " : PMIOPort  Tag=PMCPort  Port=5  Side=Right
  "c " : PMIOPort  Tag=PMCPort  Port=6  Side=Right
  connections:
  Series RLC Branch5/RConn1 -- Ground5/LConn1
  Series RLC Branch4/RConn1 -- Ground4/LConn1
  Series RLC Branch3/RConn1 -- Ground3/LConn1
  Series RLC Branch2/RConn1 -- Ground2/LConn1
  Series RLC Branch1/RConn1 -- Ground1/LConn1
  Series RLC Branch/RConn1 -- Ground/LConn1
  Series RLC Branch/LConn1 -- Config301/RConn3 -- Series RLC Branch8/RConn1 -- "c "/RConn1 -- Series RLC Branch6/RConn1
  Series RLC Branch1/LConn1 -- Config301/RConn2 -- Series RLC Branch7/RConn1 -- Series RLC Branch6/LConn1 -- "b "/RConn1
  Series RLC Branch2/LConn1 -- Config301/RConn1 -- Series RLC Branch8/LConn1 -- "a "/RConn1 -- Series RLC Branch7/LConn1
  Series RLC Branch5/LConn1 -- Config301/LConn3 -- Series RLC Branch11/RConn1 -- c/RConn1 -- Series RLC Branch10/RConn1
  Series RLC Branch4/LConn1 -- Config301/LConn2 -- Series RLC Branch10/LConn1 -- Series RLC Branch9/RConn1 -- b/RConn1
  Series RLC Branch3/LConn1 -- Config301/LConn1 -- Series RLC Branch11/LConn1 -- a/RConn1 -- Series RLC Branch9/LConn1

== system DTU_Topology_Rural/SM_Master/Cable C1 No parallel cap ==
  Config301 : spsMutualInductanceLib/Mutual Inductance  LConnTagsString=a|b|c  RConnTagsString=A|B|C  TypeOfMutual=Generalized mutual inductance  NumberOfWindings=3  SelfImpedance1=[1.1 1.1e-03]  SelfImpedance2=[ 1.1 1.1e-03]  ThreeWindings=on  SelfImpedance3=[ 1.1 1.1e-03]  MutualImpedance=[1.0 1.0e-03]  InductanceMatrix=[line_param.C1.Ls line_param.C1.Lm line_param.C1.Lm ; line_param.C1.Lm line_param.C1.Ls line_param.C1.Lm ; line_param.C1.Lm line_param.C1.Lm line_param.C1.Ls]  ResistanceMatrix=[line_param.C1.Rs line_param.C1.Rm line_param.C1.Rm ; line_param.C1.Rm line_param.C1.Rs line_param.C1.Rm ; line_param.C1.Rm line_param.C1.Rm line_param.C1.Rs]  Measurements=None
      settings: LibrarySourceBlock=sps_lib/Passives/Mutual Inductance
  Ground{,1..5} (6 alike) : spsGroundLib/Ground  LConnTagsString=a
  Series RLC Branch{,1..5} (6 alike) : spsSeriesRLCBranchLib/Series RLC Branch  LConnTagsString=__new0  RConnTagsString=__new0  BranchType=C  Resistance=1  Inductance=1e-3  SetiL0=off  InitialCurrent=0  Capacitance=line_param.C1.Cg / 2  Setx0=off  InitialVoltage=0  Measurements=None
  Series RLC Branch{6..11} (6 alike) : spsSeriesRLCBranchLib/Series RLC Branch  Commented=on  LConnTagsString=__new0  RConnTagsString=__new0  BranchType=C  Resistance=1  Inductance=1e-3  SetiL0=off  InitialCurrent=0  Capacitance=line_param.C1.Cp / 2  Setx0=off  InitialVoltage=0  Measurements=None
  a : PMIOPort  Tag=PMCPort  Side=Left
  b : PMIOPort  Tag=PMCPort  Port=2  Side=Left
  c : PMIOPort  Tag=PMCPort  Port=3  Side=Left
  "a " : PMIOPort  Tag=PMCPort  Port=4  Side=Right
  "b " : PMIOPort  Tag=PMCPort  Port=5  Side=Right
  "c " : PMIOPort  Tag=PMCPort  Port=6  Side=Right
  connections:
  Series RLC Branch5/RConn1 -- Ground5/LConn1
  Series RLC Branch4/RConn1 -- Ground4/LConn1
  Series RLC Branch3/RConn1 -- Ground3/LConn1
  Series RLC Branch2/RConn1 -- Ground2/LConn1
  Series RLC Branch1/RConn1 -- Ground1/LConn1
  Series RLC Branch/RConn1 -- Ground/LConn1
  Series RLC Branch/LConn1 -- Config301/RConn3 -- Series RLC Branch8/RConn1 -- "c "/RConn1 -- Series RLC Branch6/RConn1
  Series RLC Branch1/LConn1 -- Config301/RConn2 -- Series RLC Branch7/RConn1 -- Series RLC Branch6/LConn1 -- "b "/RConn1
  Series RLC Branch2/LConn1 -- Config301/RConn1 -- Series RLC Branch8/LConn1 -- "a "/RConn1 -- Series RLC Branch7/LConn1
  Series RLC Branch5/LConn1 -- Config301/LConn3 -- Series RLC Branch11/RConn1 -- c/RConn1 -- Series RLC Branch10/RConn1
  Series RLC Branch4/LConn1 -- Config301/LConn2 -- Series RLC Branch10/LConn1 -- Series RLC Branch9/RConn1 -- b/RConn1
  Series RLC Branch3/LConn1 -- Config301/LConn1 -- Series RLC Branch11/LConn1 -- a/RConn1 -- Series RLC Branch9/LConn1

== system DTU_Topology_Rural/SM_Master/Cable C2 No parallel cap ==
  Config301 : spsMutualInductanceLib/Mutual Inductance  LConnTagsString=a|b|c  RConnTagsString=A|B|C  TypeOfMutual=Generalized mutual inductance  NumberOfWindings=3  SelfImpedance1=[1.1 1.1e-03]  SelfImpedance2=[ 1.1 1.1e-03]  ThreeWindings=on  SelfImpedance3=[ 1.1 1.1e-03]  MutualImpedance=[1.0 1.0e-03]  InductanceMatrix=[line_param.C2.Ls line_param.C2.Lm line_param.C2.Lm ; line_param.C2.Lm line_param.C2.Ls line_param.C2.Lm ; line_param.C2.Lm line_param.C2.Lm line_param.C2.Ls]  ResistanceMatrix=[line_param.C2.Rs line_param.C2.Rm line_param.C2.Rm ; line_param.C2.Rm line_param.C2.Rs line_param.C2.Rm ; line_param.C2.Rm line_param.C2.Rm line_param.C2.Rs]  Measurements=None
      settings: LibrarySourceBlock=sps_lib/Passives/Mutual Inductance
  Ground{,1..5} (6 alike) : spsGroundLib/Ground  LConnTagsString=a
  Series RLC Branch{,1..5} (6 alike) : spsSeriesRLCBranchLib/Series RLC Branch  LConnTagsString=__new0  RConnTagsString=__new0  BranchType=C  Resistance=1  Inductance=1e-3  SetiL0=off  InitialCurrent=0  Capacitance=line_param.C2.Cg / 2  Setx0=off  InitialVoltage=0  Measurements=None
  Series RLC Branch{6..11} (6 alike) : spsSeriesRLCBranchLib/Series RLC Branch  Commented=on  LConnTagsString=__new0  RConnTagsString=__new0  BranchType=C  Resistance=1  Inductance=1e-3  SetiL0=off  InitialCurrent=0  Capacitance=line_param.C2.Cp / 2  Setx0=off  InitialVoltage=0  Measurements=None
  a : PMIOPort  Tag=PMCPort  Side=Left
  b : PMIOPort  Tag=PMCPort  Port=2  Side=Left
  c : PMIOPort  Tag=PMCPort  Port=3  Side=Left
  "a " : PMIOPort  Tag=PMCPort  Port=4  Side=Right
  "b " : PMIOPort  Tag=PMCPort  Port=5  Side=Right
  "c " : PMIOPort  Tag=PMCPort  Port=6  Side=Right
  connections:
  Series RLC Branch5/RConn1 -- Ground5/LConn1
  Series RLC Branch4/RConn1 -- Ground4/LConn1
  Series RLC Branch3/RConn1 -- Ground3/LConn1
  Series RLC Branch2/RConn1 -- Ground2/LConn1
  Series RLC Branch1/RConn1 -- Ground1/LConn1
  Series RLC Branch/RConn1 -- Ground/LConn1
  Series RLC Branch/LConn1 -- Config301/RConn3 -- Series RLC Branch8/RConn1 -- "c "/RConn1 -- Series RLC Branch6/RConn1
  Series RLC Branch1/LConn1 -- Config301/RConn2 -- Series RLC Branch7/RConn1 -- Series RLC Branch6/LConn1 -- "b "/RConn1
  Series RLC Branch2/LConn1 -- Config301/RConn1 -- Series RLC Branch8/LConn1 -- "a "/RConn1 -- Series RLC Branch7/LConn1
  Series RLC Branch5/LConn1 -- Config301/LConn3 -- Series RLC Branch11/RConn1 -- c/RConn1 -- Series RLC Branch10/RConn1
  Series RLC Branch4/LConn1 -- Config301/LConn2 -- Series RLC Branch10/LConn1 -- Series RLC Branch9/RConn1 -- b/RConn1
  Series RLC Branch3/LConn1 -- Config301/LConn1 -- Series RLC Branch11/LConn1 -- a/RConn1 -- Series RLC Branch9/LConn1

== system DTU_Topology_Rural/SM_Master/Cable E1 No parallel cap ==
  Config301 : spsMutualInductanceLib/Mutual Inductance  LConnTagsString=a|b|c  RConnTagsString=A|B|C  TypeOfMutual=Generalized mutual inductance  NumberOfWindings=3  SelfImpedance1=[1.1 1.1e-03]  SelfImpedance2=[ 1.1 1.1e-03]  ThreeWindings=on  SelfImpedance3=[ 1.1 1.1e-03]  MutualImpedance=[1.0 1.0e-03]  InductanceMatrix=[line_param.E1.Ls line_param.E1.Lm line_param.E1.Lm ; line_param.E1.Lm line_param.E1.Ls line_param.E1.Lm ; line_param.E1.Lm line_param.E1.Lm line_param.E1.Ls]  ResistanceMatrix=[line_param.E1.Rs line_param.E1.Rm line_param.E1.Rm ; line_param.E1.Rm line_param.E1.Rs line_param.E1.Rm ; line_param.E1.Rm line_param.E1.Rm line_param.E1.Rs]  Measurements=None
      settings: LibrarySourceBlock=sps_lib/Passives/Mutual Inductance
  Ground{,1..5} (6 alike) : spsGroundLib/Ground  LConnTagsString=a
  Series RLC Branch{,1..5} (6 alike) : spsSeriesRLCBranchLib/Series RLC Branch  LConnTagsString=__new0  RConnTagsString=__new0  BranchType=C  Resistance=1  Inductance=1e-3  SetiL0=off  InitialCurrent=0  Capacitance=line_param.E1.Cg / 2  Setx0=off  InitialVoltage=0  Measurements=None
  Series RLC Branch{6..11} (6 alike) : spsSeriesRLCBranchLib/Series RLC Branch  Commented=on  LConnTagsString=__new0  RConnTagsString=__new0  BranchType=C  Resistance=1  Inductance=1e-3  SetiL0=off  InitialCurrent=0  Capacitance=line_param.E1.Cp / 2  Setx0=off  InitialVoltage=0  Measurements=None
  a : PMIOPort  Tag=PMCPort  Side=Left
  b : PMIOPort  Tag=PMCPort  Port=2  Side=Left
  c : PMIOPort  Tag=PMCPort  Port=3  Side=Left
  "a " : PMIOPort  Tag=PMCPort  Port=4  Side=Right
  "b " : PMIOPort  Tag=PMCPort  Port=5  Side=Right
  "c " : PMIOPort  Tag=PMCPort  Port=6  Side=Right
  connections:
  Series RLC Branch5/RConn1 -- Ground5/LConn1
  Series RLC Branch4/RConn1 -- Ground4/LConn1
  Series RLC Branch3/RConn1 -- Ground3/LConn1
  Series RLC Branch2/RConn1 -- Ground2/LConn1
  Series RLC Branch1/RConn1 -- Ground1/LConn1
  Series RLC Branch/RConn1 -- Ground/LConn1
  Series RLC Branch/LConn1 -- Config301/RConn3 -- Series RLC Branch8/RConn1 -- "c "/RConn1 -- Series RLC Branch6/RConn1
  Series RLC Branch1/LConn1 -- Config301/RConn2 -- Series RLC Branch7/RConn1 -- Series RLC Branch6/LConn1 -- "b "/RConn1
  Series RLC Branch2/LConn1 -- Config301/RConn1 -- Series RLC Branch8/LConn1 -- "a "/RConn1 -- Series RLC Branch7/LConn1
  Series RLC Branch5/LConn1 -- Config301/LConn3 -- Series RLC Branch11/RConn1 -- c/RConn1 -- Series RLC Branch10/RConn1
  Series RLC Branch4/LConn1 -- Config301/LConn2 -- Series RLC Branch10/LConn1 -- Series RLC Branch9/RConn1 -- b/RConn1
  Series RLC Branch3/LConn1 -- Config301/LConn1 -- Series RLC Branch11/LConn1 -- a/RConn1 -- Series RLC Branch9/LConn1

== system DTU_Topology_Rural/SM_Master/Cable F1 No parallel cap ==
  Config301 : spsMutualInductanceLib/Mutual Inductance  LConnTagsString=a|b|c  RConnTagsString=A|B|C  TypeOfMutual=Generalized mutual inductance  NumberOfWindings=3  SelfImpedance1=[1.1 1.1e-03]  SelfImpedance2=[ 1.1 1.1e-03]  ThreeWindings=on  SelfImpedance3=[ 1.1 1.1e-03]  MutualImpedance=[1.0 1.0e-03]  InductanceMatrix=[line_param.F1.Ls line_param.F1.Lm line_param.F1.Lm ; line_param.F1.Lm line_param.F1.Ls line_param.F1.Lm ; line_param.F1.Lm line_param.F1.Lm line_param.F1.Ls]  ResistanceMatrix=[line_param.F1.Rs line_param.F1.Rm line_param.F1.Rm ; line_param.F1.Rm line_param.F1.Rs line_param.F1.Rm ; line_param.F1.Rm line_param.F1.Rm line_param.F1.Rs]  Measurements=None
      settings: LibrarySourceBlock=sps_lib/Passives/Mutual Inductance
  Ground{,1..5} (6 alike) : spsGroundLib/Ground  LConnTagsString=a
  Series RLC Branch{,1..5} (6 alike) : spsSeriesRLCBranchLib/Series RLC Branch  LConnTagsString=__new0  RConnTagsString=__new0  BranchType=C  Resistance=1  Inductance=1e-3  SetiL0=off  InitialCurrent=0  Capacitance=line_param.F1.Cg / 2  Setx0=off  InitialVoltage=0  Measurements=None
  Series RLC Branch{6..11} (6 alike) : spsSeriesRLCBranchLib/Series RLC Branch  Commented=on  LConnTagsString=__new0  RConnTagsString=__new0  BranchType=C  Resistance=1  Inductance=1e-3  SetiL0=off  InitialCurrent=0  Capacitance=line_param.F1.Cp / 2  Setx0=off  InitialVoltage=0  Measurements=None
  a : PMIOPort  Tag=PMCPort  Side=Left
  b : PMIOPort  Tag=PMCPort  Port=2  Side=Left
  c : PMIOPort  Tag=PMCPort  Port=3  Side=Left
  "a " : PMIOPort  Tag=PMCPort  Port=4  Side=Right
  "b " : PMIOPort  Tag=PMCPort  Port=5  Side=Right
  "c " : PMIOPort  Tag=PMCPort  Port=6  Side=Right
  connections:
  Series RLC Branch5/RConn1 -- Ground5/LConn1
  Series RLC Branch4/RConn1 -- Ground4/LConn1
  Series RLC Branch3/RConn1 -- Ground3/LConn1
  Series RLC Branch2/RConn1 -- Ground2/LConn1
  Series RLC Branch1/RConn1 -- Ground1/LConn1
  Series RLC Branch/RConn1 -- Ground/LConn1
  Series RLC Branch/LConn1 -- Config301/RConn3 -- Series RLC Branch8/RConn1 -- "c "/RConn1 -- Series RLC Branch6/RConn1
  Series RLC Branch1/LConn1 -- Config301/RConn2 -- Series RLC Branch7/RConn1 -- Series RLC Branch6/LConn1 -- "b "/RConn1
  Series RLC Branch2/LConn1 -- Config301/RConn1 -- Series RLC Branch8/LConn1 -- "a "/RConn1 -- Series RLC Branch7/LConn1
  Series RLC Branch5/LConn1 -- Config301/LConn3 -- Series RLC Branch11/RConn1 -- c/RConn1 -- Series RLC Branch10/RConn1
  Series RLC Branch4/LConn1 -- Config301/LConn2 -- Series RLC Branch10/LConn1 -- Series RLC Branch9/RConn1 -- b/RConn1
  Series RLC Branch3/LConn1 -- Config301/LConn1 -- Series RLC Branch11/LConn1 -- a/RConn1 -- Series RLC Branch9/LConn1

== system DTU_Topology_Rural/SM_Master/TrueRMS 1 ==
  In : Inport
  Mean value : spsMeanLib/Mean  Freq=fnom  Vinit=0  Ts=Ts
  Product : Product  InputSameDT=on  SaturateOnIntegerOverflow=on  OutDataTypeStr=Inherit: Same as first input
  Saturation to avoid negative sqrt : Saturate  UpperLimit=Inf  LowerLimit=0
  Sqrt : Sqrt  AlgorithmType=Newton-Raphson
  RMS : Outport  VectorParamsAs1DForOutWhenUnconnected=off
  wires:
  Saturation to avoid negative sqrt/1 -> Sqrt/1
  Mean value/1 -> Saturation to avoid negative sqrt/1
  Product/1 -> Mean value/1
  In/1 -> Product/2, Product/1
  Sqrt/1 -> RMS/1
